simulink model "Flowchart10NoActions"  (Simulink 9.0)
settings: Solver=FixedStepDiscrete  StartTime=0.0  StopTime=10.0  RelTol=1e-3  EnableMultiTasking=on
settings Model: SuppressorTable=22 serialization::archive 11 0 6 0 0 0 0 0  Creator=scaife  LastModifiedBy=ktrinh  ExtModeAutoUpdateStatusClock=off
settings DataIOCC: LimitDataPoints=on  SignalLoggingSaveFormat=ModelDataLogs  SignalLoggingName=sigsOut
settings OptimizationCC: InitFltsAndDblsToZero=on
settings DebuggingCC: SaveWithParameterizedLinksMsg=none  SignalResolutionControl=TryResolveAllWithWarning  MultiTaskDSMMsg=warning  MultiTaskCondExecSysMsg=none  StrictBusMsg=None
settings HardwareCC: TargetUnknown=on
settings SFSimCC: SimParseCustomCode=off
settings GRTTargetCC: TargetFcnLib=ansi_tfl_tmw.mat  ModelReferenceCompliant=off  ParMdlRefBuildCompliant=off  CompOptLevelCompliant=off  ConcurrentExecutionCompliant=off  CombineOutputUpdateFcns=off  MatFileLogging=off  MATLABClassNameForMDSCustomization=Simulink.SoftwareTarget.TargetSpecificTriggerConfigurationBase  GRTInterface=on

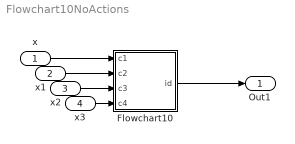
== system Flowchart10NoActions ==
  x : Inport  OutDataTypeStr=boolean
  x1 : Inport  Port=2  OutDataTypeStr=boolean
  x2 : Inport  Port=3  OutDataTypeStr=boolean
  x3 : Inport  Port=4  OutDataTypeStr=boolean
  Flowchart10 : Stateflow chart  TreatAsAtomicUnit=on
  Out1 : Outport
  wires:
  x/1 -> Flowchart10/1(c1)
  Flowchart10/1(id) -> Out1/1
  x3/1 -> Flowchart10/4(c4)
  x2/1 -> Flowchart10/3(c3)
  x1/1 -> Flowchart10/2(c2)

== stateflow chart Flowchart10 ==
  state A [parallel]
    settings: executionOrder=1
    (default) -> (junction 4) [order 1] : [c1]{id=1;}
    (default) -> (junction 5) [order 2] : [c2]{id=2;}
    A -> (junction 6) [order 2] : [c3]{id=3;}
    A -> (junction 7) [order 1] : [c4]{id=4;}
  data: c1 input boolean; c2 input boolean; c3 input boolean; c4 input boolean; id output double
